simulink model "EventCamera"  (R2024b)
settings: Solver=ode4  StartTime=0.0  StopTime=10  FixedStep=1/30  RelTol=1e-3
undefined symbols (not defined in the file or in its folder): gray, none, videoinput
libraries: imaqlib x1
settings Model: Creator=alejandromunozvazquez  LastModifiedBy=alejandromunozvazquez

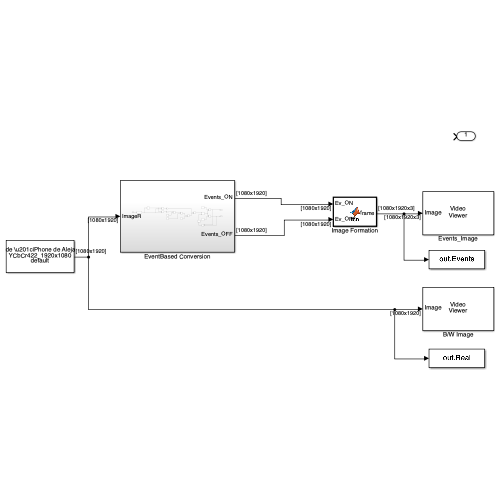
[thumbnail: Simulink's stored preview of the top-level diagram]
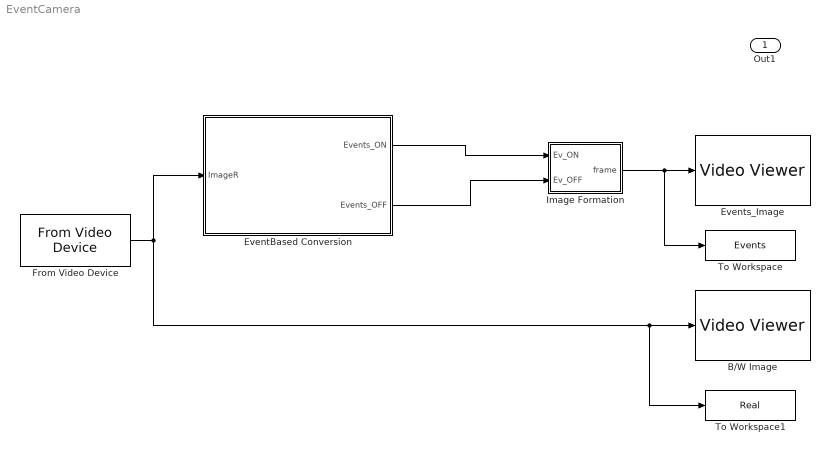
== system EventCamera ==
  B/W Image : VideoViewer  colormapValue=gray(256)  FigPos=[1 479 603 343]
  EventBased Conversion : Subsystem
  Events_Image : VideoViewer  colormapValue=gray(256)  FigPos=[1 927 601 342]
  From Video Device : imaqlib/From Video Device  DeviceMenu=macvideo 2 (C\341mara de \u201ciPhone de Alejandro\u201d)  Device=macvideo 2 (C\341mara de \u201ciPhone de Alejandro\u201d)  ObjConstructor=videoinput('macvideo', 2)  VideoFormatMenu=YCbCr422_1920x1080  VideoFormat=YCbCr422_1920x1080  VideoSource=default  ROIPosition=[0 0 1080 1920]  EnableHWTrigger=off  TriggerConfiguration=none/none  SampleTime=1/30  OutputPortsMode=One multidimensional signal  DataType=single  CanDoHWTrigger=no  ReturnedColorSpace=grayscale  BlockHandle=1621.0004  ROIWidth=1920  ROIHeight=1080  ROIColumn=0  ROIRow=0  EngXMLPath=/Applications/MATLAB_R2024b.app/toolbox/imaq/imaq/private  DevXMLPath=<binary blob, 125 chars, not shown>  EngLibPath=/Applications/MATLAB_R2024b.app/toolbox/imaq/imaqblks/imaqmex/maca64  ColorSpace=grayscale  BayerSensorAlignment=grbg  ImaqMode=off
  Image Formation : MATLAB Function  TreatAsAtomicUnit=on
  To Workspace : ToWorkspace  VariableName=Events  SaveFormat=Timeseries  SampleTime=-1
  To Workspace1 : ToWorkspace  VariableName=Real  SaveFormat=Timeseries  SampleTime=-1
  Out1 : Outport
  wires:
  EventBased Conversion/1(Events_ON) -> Image Formation/1(Ev_ON)
  EventBased Conversion/2(Events_OFF) -> Image Formation/2(Ev_OFF)
  Image Formation/1(frame) -> To Workspace/1, Events_Image/1
  From Video Device/1 -> To Workspace1/1, B/W Image/1, EventBased Conversion/1(ImageR)

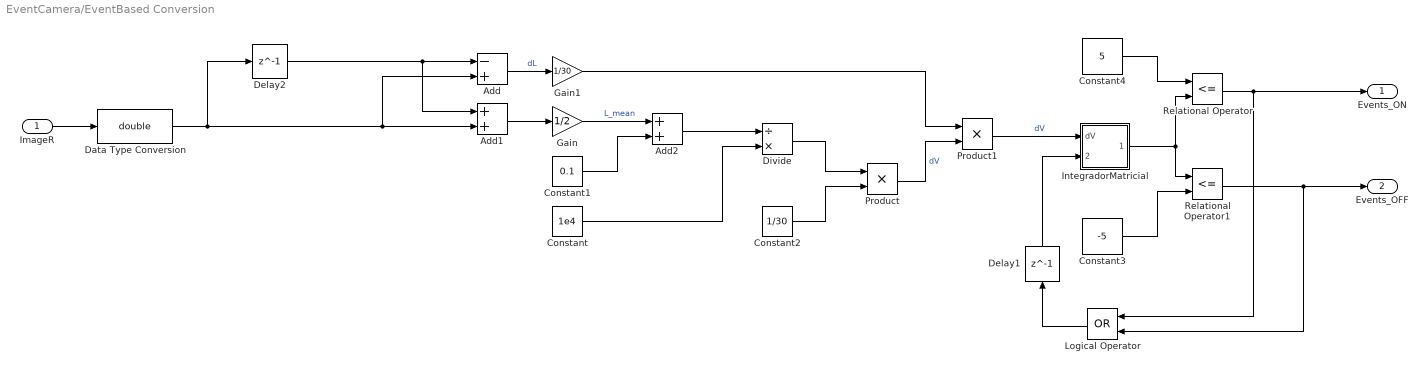
== system EventCamera/EventBased Conversion ==
  ImageR : Inport
  Add : Sum  Inputs=-+
  Add1 : Sum
  Add2 : Sum
  Constant : Constant  Value=1e4
  Constant1 : Constant  Value=0.1
  Constant2 : Constant  Value=1/30
  Constant3 : Constant  Value=-5
  Constant4 : Constant  Value=5
  Data Type Conversion : DataTypeConversion  OutDataTypeStr=double  SaturateOnIntegerOverflow=off  RndMeth=Floor
  Delay1 : Delay  DelayLength=1  InitialCondition=zeros(1080,1920)
  Delay2 : Delay  DelayLength=1  InitialCondition=zeros(1080,1920)
  Divide : Product  Inputs=/*
  Gain : Gain  Gain=1/2
  Gain1 : Gain  Gain=1/30
  IntegradorMatricial : MATLAB Function  TreatAsAtomicUnit=on
  Logical Operator : Logic  Operator=OR  AllPortsSameDT=off  OutDataTypeStr=boolean
  Product : Product
  Product1 : Product
  Relational Operator : RelationalOperator  Operator=<=  OutDataTypeStr=boolean  RndMeth=Simplest  InputSameDT=off
  Relational Operator1 : RelationalOperator  Operator=<=  OutDataTypeStr=boolean  RndMeth=Simplest  InputSameDT=off
  Events_ON : Outport
  Events_OFF : Outport  Port=2
  wires:
  ImageR/1 -> Data Type Conversion/1
  Delay2/1 -> Add1/1, Add/1
  Add1/1 -> Gain/1
  Add/1 -> Gain1/1  "dL"
  Gain/1 -> Add2/1  "L_mean"
  Constant1/1 -> Add2/2
  Add2/1 -> Divide/1
  Constant/1 -> Divide/2
  Divide/1 -> Product/1
  Constant2/1 -> Product/2
  Product/1 -> Product1/2  "dV"
  Constant4/1 -> Relational Operator/1
  Constant3/1 -> Relational Operator1/2
  IntegradorMatricial/1(dV_acc) -> Relational Operator/2, Relational Operator1/1
  Relational Operator1/1 -> Logical Operator/2, Events_OFF/1
  Relational Operator/1 -> Logical Operator/1, Events_ON/1
  Gain1/1 -> Product1/1
  Product1/1 -> IntegradorMatricial/1(dV)  "dV"
  Logical Operator/1 -> Delay1/1
  Delay1/1 -> IntegradorMatricial/2(reset)
  Data Type Conversion/1 -> Delay2/1, Add1/2, Add/2

== matlab function EventCamera/Image Formation ==
  data: Ev_ON input; frame output; Ev_OFF input
function frame = fcn(Ev_ON,Ev_OFF)

frame = uint8(zeros(1080,1920,3));

frame(:,:,1) = uint8(255*Ev_ON); 
frame(:,:,2) = uint8(255*Ev_OFF); 

end

== matlab function EventCamera/EventBased Conversion/IntegradorMatricial ==
  settings: updateMethod=DISCRETE  sampleTime=1/30
  data: dV input; dV_acc output; reset input size=[1080,1920]
function dV_acc = fcn(dV, reset)

    H = 1080;
    W = 1920;

    dV_acc = zeros(H,W);

    persistent dV_a;
    if isempty(dV_a), dV_a = zeros(H,W); end

    reset = ~reset;
    dV_a = dV_a.*reset;

    dV_a = dV_a + dV;

    dV_acc = dV_a;
